simulink model "low_pass_filter"  (R2017a)
settings: Solver=FixedStepAuto  StartTime=0.0  StopTime=4  FixedStep=1e-4  RelTol=1e-3
values from neighbouring files (symbols this model uses):
  filter_pole = 30    [Init_SNR_sim.m]
settings Model: Creator=ignacio  LastModifiedBy=ignacio

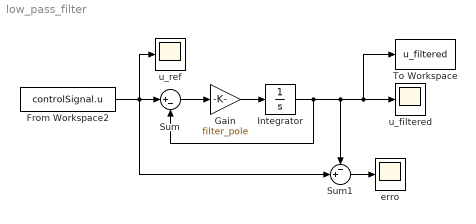
== system low_pass_filter ==
  From Workspace2 : FromWorkspace  VariableName=controlSignal.u  SampleTime=0
  Gain : Gain  Gain=filter_pole
  Integrator : Integrator
  Sum : Sum  Inputs=|+-
  Sum1 : Sum  Inputs=-+|
  To Workspace : ToWorkspace  VariableName=u_filtered  SaveFormat=Timeseries  SampleTime=-1
  erro : Scope
  u_filtered : Scope
  u_ref : Scope
  wires:
  Sum1/1 -> erro/1
  Integrator/1 -> To Workspace/1, u_filtered/1, Sum1/1, Sum/2
  From Workspace2/1 -> Sum1/2, u_ref/1, Sum/1
  Sum/1 -> Gain/1
  Gain/1 -> Integrator/1
